simulink model "SecRwLtStHdrstFwdBkwdTrgtPosSelc"  (R2018b)
settings: Solver=FixedStepDiscrete  StartTime=0.0  StopTime=10.0  FixedStep=0.01  RelTol=1e-3
undefined symbols (not defined in the file or in its folder): KeSMSw4SAcsMd21SecRwLtStHdrstFrwdBkwdPos_Val, KeSMSw4SAcsMd21SecRwLtStHdrstFrwdBkwdPosMax_Val, KeSMSw4SAcsMd21SecRwLtStHdrstFrwdBkwdPosMin_Val, KeSMSw4SAcsMd22SecRwLtStHdrstFrwdBkwdPos_Val, KeSMSw4SAcsMd22SecRwLtStHdrstFrwdBkwdPosMax_Val, KeSMSw4SAcsMd22SecRwLtStHdrstFrwdBkwdPosMin_Val, KeSMSw4SAcsMd25SecRwLtStHdrstFrwdBkwdPos_Val, KeSMSw4SAcsMd25SecRwLtStHdrstFrwdBkwdPosMax_Val, KeSMSw4SAcsMd25SecRwLtStHdrstFrwdBkwdPosMin_Val, KeSMSw4SAcsMd26SecRwLtStHdrstFrwdBkwdPos_Val, KeSMSw4SAcsMd26SecRwLtStHdrstFrwdBkwdPosMax_Val, KeSMSw4SAcsMd26SecRwLtStHdrstFrwdBkwdPosMin_Val, KeSMSw4sLyingMDSecRwLtStHdrstFrwdBkwdnwdPos_160_Val, KeSMSw4sLyingMDSecRwLtStHdrstFrwdBkwdnwdPos_165_Val, KeSMSw4sLyingMDSecRwLtStHdrstFrwdBkwdnwdPos_170_Val, KeSMSw4sLyingMDSecRwLtStHdrstFrwdBkwdnwdPos_175_Val, KeSMSw4sLyingMDSecRwLtStHdrstFrwdBkwdnwdPos_180_Val, KeSMSw4sLyingMDSecRwLtStHdrstFrwdBkwdnwdPos_Below160_Val, KeSMSw4sLyingMDSecRwLtStHdrstFrwdBkwdnwdPos_Over180_Val, KeSMSw4sLyingMDSecRwLtStHdrstFrwdBkwdnwdPosMax_160_Val, KeSMSw4sLyingMDSecRwLtStHdrstFrwdBkwdnwdPosMax_165_Val, KeSMSw4sLyingMDSecRwLtStHdrstFrwdBkwdnwdPosMax_170_Val, KeSMSw4sLyingMDSecRwLtStHdrstFrwdBkwdnwdPosMax_175_Val, KeSMSw4sLyingMDSecRwLtStHdrstFrwdBkwdnwdPosMax_180_Val, KeSMSw4sLyingMDSecRwLtStHdrstFrwdBkwdnwdPosMax_Below160_Val, KeSMSw4sLyingMDSecRwLtStHdrstFrwdBkwdnwdPosMax_Over180_Val, KeSMSw4sLyingMDSecRwLtStHdrstFrwdBkwdnwdPosMin_160_Val, KeSMSw4sLyingMDSecRwLtStHdrstFrwdBkwdnwdPosMin_165_Val, KeSMSw4sLyingMDSecRwLtStHdrstFrwdBkwdnwdPosMin_170_Val, KeSMSw4sLyingMDSecRwLtStHdrstFrwdBkwdnwdPosMin_175_Val, KeSMSw4sLyingMDSecRwLtStHdrstFrwdBkwdnwdPosMin_180_Val, KeSMSw4sLyingMDSecRwLtStHdrstFrwdBkwdnwdPosMin_Below160_Val, KeSMSw4sLyingMDSecRwLtStHdrstFrwdBkwdnwdPosMin_Over180_Val, KeSMSw4sRecoveryMDSecRwLtStHdrstFrwdBkwdPos_160_Val, KeSMSw4sRecoveryMDSecRwLtStHdrstFrwdBkwdPos_165_Val, KeSMSw4sRecoveryMDSecRwLtStHdrstFrwdBkwdPos_170_Val, KeSMSw4sRecoveryMDSecRwLtStHdrstFrwdBkwdPos_175_Val, KeSMSw4sRecoveryMDSecRwLtStHdrstFrwdBkwdPos_180_Val, KeSMSw4sRecoveryMDSecRwLtStHdrstFrwdBkwdPos_Below160_Val, KeSMSw4sRecoveryMDSecRwLtStHdrstFrwdBkwdPos_Over180_Val, KeSMSw4sRecoveryMDSecRwLtStHdrstFrwdBkwdPosMax_160_Val, KeSMSw4sRecoveryMDSecRwLtStHdrstFrwdBkwdPosMax_165_Val, KeSMSw4sRecoveryMDSecRwLtStHdrstFrwdBkwdPosMax_170_Val, KeSMSw4sRecoveryMDSecRwLtStHdrstFrwdBkwdPosMax_175_Val, KeSMSw4sRecoveryMDSecRwLtStHdrstFrwdBkwdPosMax_180_Val, KeSMSw4sRecoveryMDSecRwLtStHdrstFrwdBkwdPosMax_Below160_Val, KeSMSw4sRecoveryMDSecRwLtStHdrstFrwdBkwdPosMax_Over180_Val, KeSMSw4sRecoveryMDSecRwLtStHdrstFrwdBkwdPosMin_160_Val, KeSMSw4sRecoveryMDSecRwLtStHdrstFrwdBkwdPosMin_165_Val, KeSMSw4sRecoveryMDSecRwLtStHdrstFrwdBkwdPosMin_170_Val, KeSMSw4sRecoveryMDSecRwLtStHdrstFrwdBkwdPosMin_175_Val, KeSMSw4sRecoveryMDSecRwLtStHdrstFrwdBkwdPosMin_180_Val, KeSMSw4sRecoveryMDSecRwLtStHdrstFrwdBkwdPosMin_Below160_Val, KeSMSw4sRecoveryMDSecRwLtStHdrstFrwdBkwdPosMin_Over180_Val, KeSMSw4sVIPMDSecRwLtStHdrstFrwdBkwdPos_160_Val, KeSMSw4sVIPMDSecRwLtStHdrstFrwdBkwdPos_165_Val, KeSMSw4sVIPMDSecRwLtStHdrstFrwdBkwdPos_170_Val, KeSMSw4sVIPMDSecRwLtStHdrstFrwdBkwdPos_175_Val, KeSMSw4sVIPMDSecRwLtStHdrstFrwdBkwdPos_180_Val, KeSMSw4sVIPMDSecRwLtStHdrstFrwdBkwdPos_Below160_Val ... (+15)
libraries: TrgtPosSelcLib x7
settings Model: ModifiedHistory=2023.8.1 V2.0.0 CR401790 增加模式21-26  Creator=sn2xws  LastModifiedBy=sn2xws
settings DataIOCC: SaveFormat=StructureWithTime
settings OptimizationCC: DefaultParameterBehavior=Inlined  EnhancedBackFolding=on  PassReuseOutputArgsAs=Individual arguments  ZeroExternalMemoryAtStartup=off  ZeroInternalMemoryAtStartup=off  OptimizeBlockOrder=speed  DifferentSizesBufferReuse=on  OptimizationCustomize=off
settings DebuggingCC: ParameterTunabilityLossMsg=error
settings ModelReferenceCC: ModelReferenceNumInstancesAllowed=Single
settings SFSimCC: MATLABDynamicMemAlloc=off
settings RTWCC: SystemTargetFile=autosar.tlc  GenCodeOnly=on  TemplateMakefile=ert_default_tmf  Description=AUTOSAR  GenerateReport=on  IncludeHyperlinkInReport=on  LaunchReport=on  GenerateTraceInfo=on  GenerateTraceReport=on  GenerateTraceReportSl=on  GenerateTraceReportSf=on  GenerateTraceReportEml=on  GenerateCodeMetricsReport=on
settings CodeAppCC: ForceParamTrailComments=on  IgnoreCustomStorageClasses=off  OperatorAnnotations=on  SimulinkDataObjDesc=on  SFDataObjDesc=on  InsertBlockDesc=on
settings STFCustomTargetCC: TargetLangStandard=C99 (ISO)  MultiwordLength=256  ParMdlRefBuildCompliant=on  CompOptLevelCompliant=on  IncludeMdlTerminateFcn=off  CombineOutputUpdateFcns=on  SuppressErrorStatus=on  ERTCustomFileBanners=on  SupportNonFinite=off  SupportComplex=off  SupportContinuousTime=off  SupportNonInlinedSFcns=off  RemoveResetFunc=on  MATLABClassNameForMDSCustomization=Simulink.SoftwareTarget.ERTCustomization  AutosarCompliant=on  UseToolchainInfoCompliant=on  LookupTableObjectStructAxisOrder=2,1,3,4,...  LUTObjectStructOrderEvenSpacing=Size,Table,Breakpoints  SystemTargetFile=autosar.tlc
settings ERTTargetCC: TargetLangStandard=C99 (ISO)  ConcurrentExecutionCompliant=off  IncludeMdlTerminateFcn=off  SuppressErrorStatus=on  SupportNonFinite=off  SupportComplex=off  ModelStepFunctionPrototypeControlCompliant=off  CPPClassGenCompliant=off  AutosarCompliant=on  LookupTableObjectStructAxisOrder=2,1,3,4,...  LUTObjectStructOrderEvenSpacing=Size,Table,Breakpoints  InlinedParameterPlacement=NonHierarchical  ERTCustomFileTemplate=example_file_process.tlc  ERTFilePackagingFormat=Compact

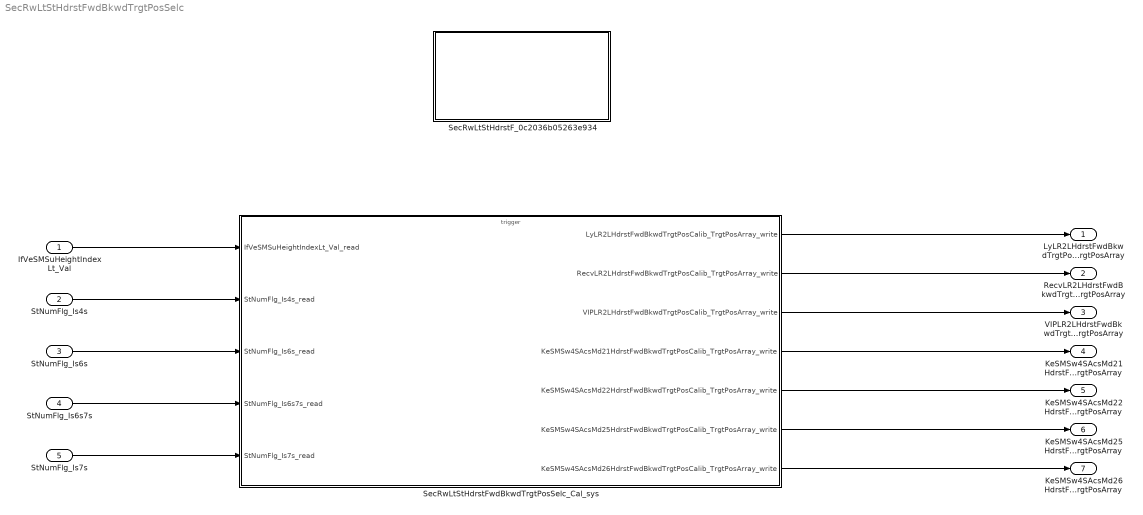
== system SecRwLtStHdrstFwdBkwdTrgtPosSelc ==
  IfVeSMSuHeightIndexLt_Val : Inport  Description=|  OutDataTypeStr=uint8  PortDimensions=1
      | 0：under 160
      | 1：160
      | 2：165
      | 3：170
      | 4：175
      | 5：180
      | 6：over 180
  StNumFlg_Is4s : Inport  Port=2  OutDataTypeStr=boolean  PortDimensions=1
  StNumFlg_Is6s : Inport  Port=3  OutDataTypeStr=boolean  PortDimensions=1
  StNumFlg_Is6s7s : Inport  Port=4  OutDataTypeStr=boolean  PortDimensions=1
  StNumFlg_Is7s : Inport  Port=5  OutDataTypeStr=boolean  PortDimensions=1
  SecRwLtStHdrstF_0c2036b05263e934 : Subsystem
  SecRwLtStHdrstFwdBkwdTrgtPosSelc_Cal_sys : Subsystem
  LyLR2LHdrstFwdBkwdTrgtPosCalib_TrgtPosArray : Outport  Description=|  OutDataTypeStr=uint16  PortDimensions=3
      | 0:Pos
      | 1:Max
      | 2:Min
  RecvLR2LHdrstFwdBkwdTrgtPosCalib_TrgtPosArray : Outport  Description=|  Port=2  OutDataTypeStr=uint16  PortDimensions=3
      | 0:Pos
      | 1:Max
      | 2:Min
  VIPLR2LHdrstFwdBkwdTrgtPosCalib_TrgtPosArray : Outport  Description=|  Port=3  OutDataTypeStr=uint16  PortDimensions=3
      | 0:Pos
      | 1:Max
      | 2:Min
  KeSMSw4SAcsMd21HdrstFwdBkwdTrgtPosCalib_TrgtPosArray : Outport  Description=|  Port=4  OutDataTypeStr=uint16  PortDimensions=3
      | 0:Pos
      | 1:Max
      | 2:Min
  KeSMSw4SAcsMd22HdrstFwdBkwdTrgtPosCalib_TrgtPosArray : Outport  Description=|  Port=5  OutDataTypeStr=uint16  PortDimensions=3
      | 0:Pos
      | 1:Max
      | 2:Min
  KeSMSw4SAcsMd25HdrstFwdBkwdTrgtPosCalib_TrgtPosArray : Outport  Description=|  Port=6  OutDataTypeStr=uint16  PortDimensions=3
      | 0:Pos
      | 1:Max
      | 2:Min
  KeSMSw4SAcsMd26HdrstFwdBkwdTrgtPosCalib_TrgtPosArray : Outport  Description=|  Port=7  OutDataTypeStr=uint16  PortDimensions=3
      | 0:Pos
      | 1:Max
      | 2:Min
  wires:
  IfVeSMSuHeightIndexLt_Val/1 -> SecRwLtStHdrstFwdBkwdTrgtPosSelc_Cal_sys/1(IfVeSMSuHeightIndexLt_Val_read)
  StNumFlg_Is4s/1 -> SecRwLtStHdrstFwdBkwdTrgtPosSelc_Cal_sys/2(StNumFlg_Is4s_read)
  StNumFlg_Is6s/1 -> SecRwLtStHdrstFwdBkwdTrgtPosSelc_Cal_sys/3(StNumFlg_Is6s_read)
  StNumFlg_Is6s7s/1 -> SecRwLtStHdrstFwdBkwdTrgtPosSelc_Cal_sys/4(StNumFlg_Is6s7s_read)
  StNumFlg_Is7s/1 -> SecRwLtStHdrstFwdBkwdTrgtPosSelc_Cal_sys/5(StNumFlg_Is7s_read)
  SecRwLtStHdrstFwdBkwdTrgtPosSelc_Cal_sys/1(LyLR2LHdrstFwdBkwdTrgtPosCalib_TrgtPosArray_write) -> LyLR2LHdrstFwdBkwdTrgtPosCalib_TrgtPosArray/1
  SecRwLtStHdrstFwdBkwdTrgtPosSelc_Cal_sys/2(RecvLR2LHdrstFwdBkwdTrgtPosCalib_TrgtPosArray_write) -> RecvLR2LHdrstFwdBkwdTrgtPosCalib_TrgtPosArray/1
  SecRwLtStHdrstFwdBkwdTrgtPosSelc_Cal_sys/3(VIPLR2LHdrstFwdBkwdTrgtPosCalib_TrgtPosArray_write) -> VIPLR2LHdrstFwdBkwdTrgtPosCalib_TrgtPosArray/1
  SecRwLtStHdrstFwdBkwdTrgtPosSelc_Cal_sys/4(KeSMSw4SAcsMd21HdrstFwdBkwdTrgtPosCalib_TrgtPosArray_write) -> KeSMSw4SAcsMd21HdrstFwdBkwdTrgtPosCalib_TrgtPosArray/1
  SecRwLtStHdrstFwdBkwdTrgtPosSelc_Cal_sys/5(KeSMSw4SAcsMd22HdrstFwdBkwdTrgtPosCalib_TrgtPosArray_write) -> KeSMSw4SAcsMd22HdrstFwdBkwdTrgtPosCalib_TrgtPosArray/1
  SecRwLtStHdrstFwdBkwdTrgtPosSelc_Cal_sys/6(KeSMSw4SAcsMd25HdrstFwdBkwdTrgtPosCalib_TrgtPosArray_write) -> KeSMSw4SAcsMd25HdrstFwdBkwdTrgtPosCalib_TrgtPosArray/1
  SecRwLtStHdrstFwdBkwdTrgtPosSelc_Cal_sys/7(KeSMSw4SAcsMd26HdrstFwdBkwdTrgtPosCalib_TrgtPosArray_write) -> KeSMSw4SAcsMd26HdrstFwdBkwdTrgtPosCalib_TrgtPosArray/1

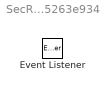
== system SecRwLtStHdrstFwdBkwdTrgtPosSelc/SecRwLtStHdrstF_0c2036b05263e934 ==
  Event Listener : EventListener  EventName=reset

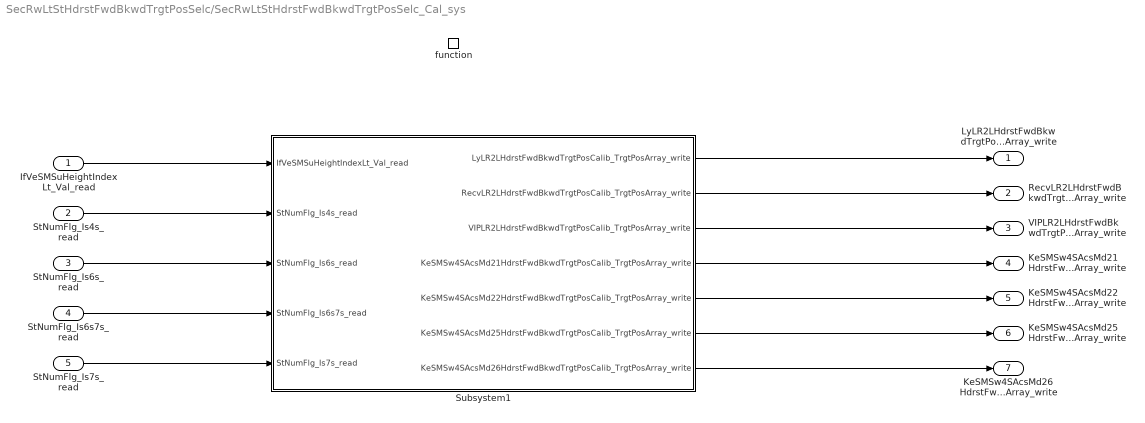
== system SecRwLtStHdrstFwdBkwdTrgtPosSelc/SecRwLtStHdrstFwdBkwdTrgtPosSelc_Cal_sys ==
  IfVeSMSuHeightIndexLt_Val_read : Inport
  StNumFlg_Is4s_read : Inport  Port=2
  StNumFlg_Is6s_read : Inport  Port=3
  StNumFlg_Is6s7s_read : Inport  Port=4
  StNumFlg_Is7s_read : Inport  Port=5
  function : TriggerPort  TriggerType=function-call  IsSimulinkFunction=on  FunctionName=SecRwLtStHdrstFwdBkwdTrgtPosSelc_Cal  VariantControl=(inherit)
  Subsystem1 : Subsystem
  LyLR2LHdrstFwdBkwdTrgtPosCalib_TrgtPosArray_write : Outport
      settings: EnsureOutportIsVirtual=on
  RecvLR2LHdrstFwdBkwdTrgtPosCalib_TrgtPosArray_write : Outport  Port=2
      settings: EnsureOutportIsVirtual=on
  VIPLR2LHdrstFwdBkwdTrgtPosCalib_TrgtPosArray_write : Outport  Port=3
      settings: EnsureOutportIsVirtual=on
  KeSMSw4SAcsMd21HdrstFwdBkwdTrgtPosCalib_TrgtPosArray_write : Outport  Port=4
      settings: EnsureOutportIsVirtual=on
  KeSMSw4SAcsMd22HdrstFwdBkwdTrgtPosCalib_TrgtPosArray_write : Outport  Port=5
      settings: EnsureOutportIsVirtual=on
  KeSMSw4SAcsMd25HdrstFwdBkwdTrgtPosCalib_TrgtPosArray_write : Outport  Port=6
      settings: EnsureOutportIsVirtual=on
  KeSMSw4SAcsMd26HdrstFwdBkwdTrgtPosCalib_TrgtPosArray_write : Outport  Port=7
      settings: EnsureOutportIsVirtual=on
  wires:
  Subsystem1/1(LyLR2LHdrstFwdBkwdTrgtPosCalib_TrgtPosArray_write) -> LyLR2LHdrstFwdBkwdTrgtPosCalib_TrgtPosArray_write/1
  Subsystem1/2(RecvLR2LHdrstFwdBkwdTrgtPosCalib_TrgtPosArray_write) -> RecvLR2LHdrstFwdBkwdTrgtPosCalib_TrgtPosArray_write/1
  Subsystem1/3(VIPLR2LHdrstFwdBkwdTrgtPosCalib_TrgtPosArray_write) -> VIPLR2LHdrstFwdBkwdTrgtPosCalib_TrgtPosArray_write/1
  Subsystem1/4(KeSMSw4SAcsMd21HdrstFwdBkwdTrgtPosCalib_TrgtPosArray_write) -> KeSMSw4SAcsMd21HdrstFwdBkwdTrgtPosCalib_TrgtPosArray_write/1
  Subsystem1/5(KeSMSw4SAcsMd22HdrstFwdBkwdTrgtPosCalib_TrgtPosArray_write) -> KeSMSw4SAcsMd22HdrstFwdBkwdTrgtPosCalib_TrgtPosArray_write/1
  Subsystem1/6(KeSMSw4SAcsMd25HdrstFwdBkwdTrgtPosCalib_TrgtPosArray_write) -> KeSMSw4SAcsMd25HdrstFwdBkwdTrgtPosCalib_TrgtPosArray_write/1
  Subsystem1/7(KeSMSw4SAcsMd26HdrstFwdBkwdTrgtPosCalib_TrgtPosArray_write) -> KeSMSw4SAcsMd26HdrstFwdBkwdTrgtPosCalib_TrgtPosArray_write/1
  StNumFlg_Is4s_read/1 -> Subsystem1/2(StNumFlg_Is4s_read)
  StNumFlg_Is6s_read/1 -> Subsystem1/3(StNumFlg_Is6s_read)
  IfVeSMSuHeightIndexLt_Val_read/1 -> Subsystem1/1(IfVeSMSuHeightIndexLt_Val_read)
  StNumFlg_Is6s7s_read/1 -> Subsystem1/4(StNumFlg_Is6s7s_read)
  StNumFlg_Is7s_read/1 -> Subsystem1/5(StNumFlg_Is7s_read)

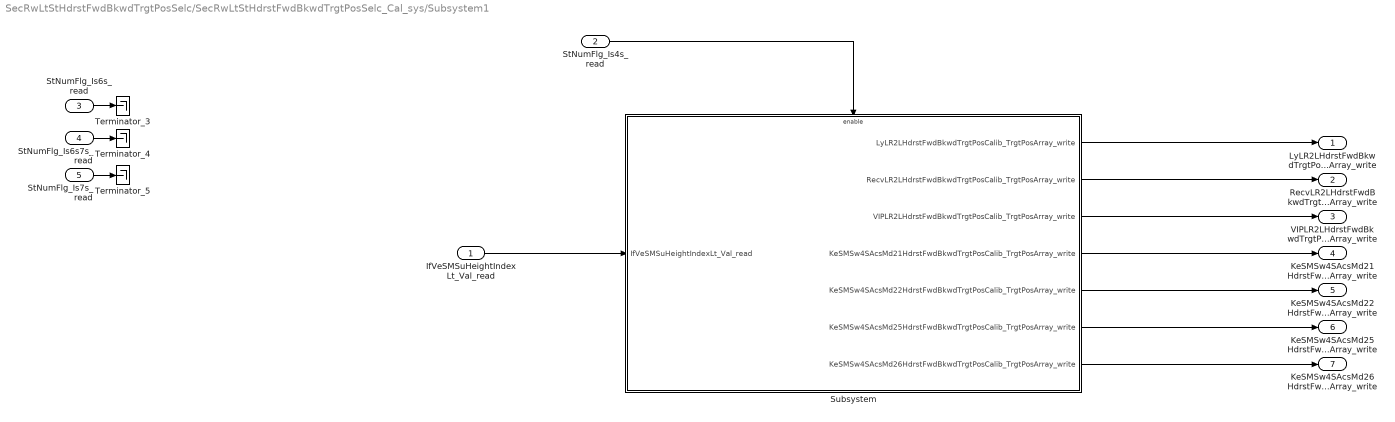
== system SecRwLtStHdrstFwdBkwdTrgtPosSelc/SecRwLtStHdrstFwdBkwdTrgtPosSelc_Cal_sys/Subsystem1 ==
  IfVeSMSuHeightIndexLt_Val_read : Inport
  StNumFlg_Is4s_read : Inport  Port=2
  StNumFlg_Is6s_read : Inport  Port=3
  StNumFlg_Is6s7s_read : Inport  Port=4
  StNumFlg_Is7s_read : Inport  Port=5
  Subsystem : Subsystem
  Terminator_3 : Terminator
  Terminator_4 : Terminator
  Terminator_5 : Terminator
  LyLR2LHdrstFwdBkwdTrgtPosCalib_TrgtPosArray_write : Outport
      settings: EnsureOutportIsVirtual=on
  RecvLR2LHdrstFwdBkwdTrgtPosCalib_TrgtPosArray_write : Outport  Port=2
      settings: EnsureOutportIsVirtual=on
  VIPLR2LHdrstFwdBkwdTrgtPosCalib_TrgtPosArray_write : Outport  Port=3
      settings: EnsureOutportIsVirtual=on
  KeSMSw4SAcsMd21HdrstFwdBkwdTrgtPosCalib_TrgtPosArray_write : Outport  Port=4
      settings: EnsureOutportIsVirtual=on
  KeSMSw4SAcsMd22HdrstFwdBkwdTrgtPosCalib_TrgtPosArray_write : Outport  Port=5
      settings: EnsureOutportIsVirtual=on
  KeSMSw4SAcsMd25HdrstFwdBkwdTrgtPosCalib_TrgtPosArray_write : Outport  Port=6
      settings: EnsureOutportIsVirtual=on
  KeSMSw4SAcsMd26HdrstFwdBkwdTrgtPosCalib_TrgtPosArray_write : Outport  Port=7
      settings: EnsureOutportIsVirtual=on
  wires:
  Subsystem/2(RecvLR2LHdrstFwdBkwdTrgtPosCalib_TrgtPosArray_write) -> RecvLR2LHdrstFwdBkwdTrgtPosCalib_TrgtPosArray_write/1
  Subsystem/1(LyLR2LHdrstFwdBkwdTrgtPosCalib_TrgtPosArray_write) -> LyLR2LHdrstFwdBkwdTrgtPosCalib_TrgtPosArray_write/1
  StNumFlg_Is4s_read/1 -> Subsystem/Enable
  IfVeSMSuHeightIndexLt_Val_read/1 -> Subsystem/1(IfVeSMSuHeightIndexLt_Val_read)
  Subsystem/3(VIPLR2LHdrstFwdBkwdTrgtPosCalib_TrgtPosArray_write) -> VIPLR2LHdrstFwdBkwdTrgtPosCalib_TrgtPosArray_write/1
  StNumFlg_Is7s_read/1 -> Terminator_5/1
  StNumFlg_Is6s7s_read/1 -> Terminator_4/1
  StNumFlg_Is6s_read/1 -> Terminator_3/1
  Subsystem/7(KeSMSw4SAcsMd26HdrstFwdBkwdTrgtPosCalib_TrgtPosArray_write) -> KeSMSw4SAcsMd26HdrstFwdBkwdTrgtPosCalib_TrgtPosArray_write/1
  Subsystem/6(KeSMSw4SAcsMd25HdrstFwdBkwdTrgtPosCalib_TrgtPosArray_write) -> KeSMSw4SAcsMd25HdrstFwdBkwdTrgtPosCalib_TrgtPosArray_write/1
  Subsystem/5(KeSMSw4SAcsMd22HdrstFwdBkwdTrgtPosCalib_TrgtPosArray_write) -> KeSMSw4SAcsMd22HdrstFwdBkwdTrgtPosCalib_TrgtPosArray_write/1
  Subsystem/4(KeSMSw4SAcsMd21HdrstFwdBkwdTrgtPosCalib_TrgtPosArray_write) -> KeSMSw4SAcsMd21HdrstFwdBkwdTrgtPosCalib_TrgtPosArray_write/1

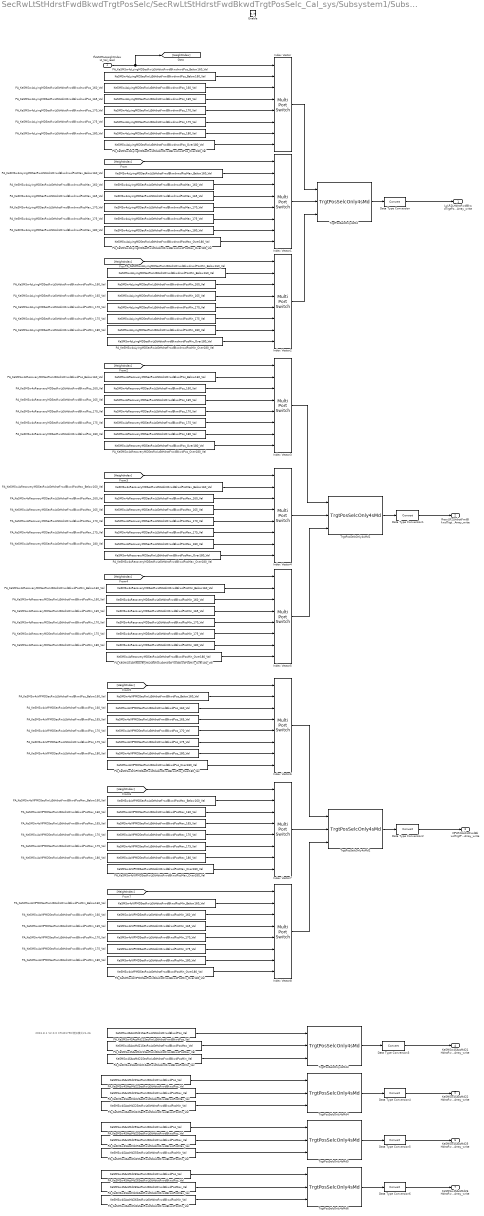
== system SecRwLtStHdrstFwdBkwdTrgtPosSelc/SecRwLtStHdrstFwdBkwdTrgtPosSelc_Cal_sys/Subsystem1/Subsystem ==
  note: 2023.8.1 V2.0.0 CR401790 增加模式21-26
  IfVeSMSuHeightIndexLt_Val_read : Inport
  Enable : EnablePort
  Data Type Conversion{,1..6} (7 alike) : DataTypeConversion
  Index Vector{,1..8} (9 alike) : MultiPortSwitch  DataPortOrder=Zero-based contiguous  Inputs=7  zeroidx=on
  PA_KeSMSw4SAcsMd21SecRwLtStHdrstFrwdBkwdPosMax_Val : Constant  Value=KeSMSw4SAcsMd21SecRwLtStHdrstFrwdBkwdPosMax_Val
  PA_KeSMSw4SAcsMd21SecRwLtStHdrstFrwdBkwdPosMin_Val : Constant  Value=KeSMSw4SAcsMd21SecRwLtStHdrstFrwdBkwdPosMin_Val
  PA_KeSMSw4SAcsMd21SecRwLtStHdrstFrwdBkwdPos_Val : Constant  Value=KeSMSw4SAcsMd21SecRwLtStHdrstFrwdBkwdPos_Val
  PA_KeSMSw4SAcsMd22SecRwLtStHdrstFrwdBkwdPosMax_Val : Constant  Value=KeSMSw4SAcsMd22SecRwLtStHdrstFrwdBkwdPosMax_Val
  PA_KeSMSw4SAcsMd22SecRwLtStHdrstFrwdBkwdPosMin_Val : Constant  Value=KeSMSw4SAcsMd22SecRwLtStHdrstFrwdBkwdPosMin_Val
  PA_KeSMSw4SAcsMd22SecRwLtStHdrstFrwdBkwdPos_Val : Constant  Value=KeSMSw4SAcsMd22SecRwLtStHdrstFrwdBkwdPos_Val
  PA_KeSMSw4SAcsMd25SecRwLtStHdrstFrwdBkwdPosMax_Val : Constant  Value=KeSMSw4SAcsMd25SecRwLtStHdrstFrwdBkwdPosMax_Val
  PA_KeSMSw4SAcsMd25SecRwLtStHdrstFrwdBkwdPosMin_Val : Constant  Value=KeSMSw4SAcsMd25SecRwLtStHdrstFrwdBkwdPosMin_Val
  PA_KeSMSw4SAcsMd25SecRwLtStHdrstFrwdBkwdPos_Val : Constant  Value=KeSMSw4SAcsMd25SecRwLtStHdrstFrwdBkwdPos_Val
  PA_KeSMSw4SAcsMd26SecRwLtStHdrstFrwdBkwdPosMax_Val : Constant  Value=KeSMSw4SAcsMd26SecRwLtStHdrstFrwdBkwdPosMax_Val
  PA_KeSMSw4SAcsMd26SecRwLtStHdrstFrwdBkwdPosMin_Val : Constant  Value=KeSMSw4SAcsMd26SecRwLtStHdrstFrwdBkwdPosMin_Val
  PA_KeSMSw4SAcsMd26SecRwLtStHdrstFrwdBkwdPos_Val : Constant  Value=KeSMSw4SAcsMd26SecRwLtStHdrstFrwdBkwdPos_Val
  PA_KeSMSw4sLyingMDSecRwLtStHdrstFrwdBkwdnwdPosMax_160_Val : Constant  Value=KeSMSw4sLyingMDSecRwLtStHdrstFrwdBkwdnwdPosMax_160_Val
  PA_KeSMSw4sLyingMDSecRwLtStHdrstFrwdBkwdnwdPosMax_165_Val : Constant  Value=KeSMSw4sLyingMDSecRwLtStHdrstFrwdBkwdnwdPosMax_165_Val
  PA_KeSMSw4sLyingMDSecRwLtStHdrstFrwdBkwdnwdPosMax_170_Val : Constant  Value=KeSMSw4sLyingMDSecRwLtStHdrstFrwdBkwdnwdPosMax_170_Val
  PA_KeSMSw4sLyingMDSecRwLtStHdrstFrwdBkwdnwdPosMax_175_Val : Constant  Value=KeSMSw4sLyingMDSecRwLtStHdrstFrwdBkwdnwdPosMax_175_Val
  PA_KeSMSw4sLyingMDSecRwLtStHdrstFrwdBkwdnwdPosMax_180_Val : Constant  Value=KeSMSw4sLyingMDSecRwLtStHdrstFrwdBkwdnwdPosMax_180_Val
  PA_KeSMSw4sLyingMDSecRwLtStHdrstFrwdBkwdnwdPosMax_Below160_Val : Constant  Value=KeSMSw4sLyingMDSecRwLtStHdrstFrwdBkwdnwdPosMax_Below160_Val
  PA_KeSMSw4sLyingMDSecRwLtStHdrstFrwdBkwdnwdPosMax_Over180_Val : Constant  Value=KeSMSw4sLyingMDSecRwLtStHdrstFrwdBkwdnwdPosMax_Over180_Val
  PA_KeSMSw4sLyingMDSecRwLtStHdrstFrwdBkwdnwdPosMin_160_Val : Constant  Value=KeSMSw4sLyingMDSecRwLtStHdrstFrwdBkwdnwdPosMin_160_Val
  PA_KeSMSw4sLyingMDSecRwLtStHdrstFrwdBkwdnwdPosMin_165_Val : Constant  Value=KeSMSw4sLyingMDSecRwLtStHdrstFrwdBkwdnwdPosMin_165_Val
  PA_KeSMSw4sLyingMDSecRwLtStHdrstFrwdBkwdnwdPosMin_170_Val : Constant  Value=KeSMSw4sLyingMDSecRwLtStHdrstFrwdBkwdnwdPosMin_170_Val
  PA_KeSMSw4sLyingMDSecRwLtStHdrstFrwdBkwdnwdPosMin_175_Val : Constant  Value=KeSMSw4sLyingMDSecRwLtStHdrstFrwdBkwdnwdPosMin_175_Val
  PA_KeSMSw4sLyingMDSecRwLtStHdrstFrwdBkwdnwdPosMin_180_Val : Constant  Value=KeSMSw4sLyingMDSecRwLtStHdrstFrwdBkwdnwdPosMin_180_Val
  PA_KeSMSw4sLyingMDSecRwLtStHdrstFrwdBkwdnwdPosMin_Below160_Val : Constant  Value=KeSMSw4sLyingMDSecRwLtStHdrstFrwdBkwdnwdPosMin_Below160_Val
  PA_KeSMSw4sLyingMDSecRwLtStHdrstFrwdBkwdnwdPosMin_Over180_Val : Constant  Value=KeSMSw4sLyingMDSecRwLtStHdrstFrwdBkwdnwdPosMin_Over180_Val
  PA_KeSMSw4sLyingMDSecRwLtStHdrstFrwdBkwdnwdPos_160_Val : Constant  Value=KeSMSw4sLyingMDSecRwLtStHdrstFrwdBkwdnwdPos_160_Val
  PA_KeSMSw4sLyingMDSecRwLtStHdrstFrwdBkwdnwdPos_165_Val : Constant  Value=KeSMSw4sLyingMDSecRwLtStHdrstFrwdBkwdnwdPos_165_Val
  PA_KeSMSw4sLyingMDSecRwLtStHdrstFrwdBkwdnwdPos_170_Val : Constant  Value=KeSMSw4sLyingMDSecRwLtStHdrstFrwdBkwdnwdPos_170_Val
  PA_KeSMSw4sLyingMDSecRwLtStHdrstFrwdBkwdnwdPos_175_Val : Constant  Value=KeSMSw4sLyingMDSecRwLtStHdrstFrwdBkwdnwdPos_175_Val
  PA_KeSMSw4sLyingMDSecRwLtStHdrstFrwdBkwdnwdPos_180_Val : Constant  Value=KeSMSw4sLyingMDSecRwLtStHdrstFrwdBkwdnwdPos_180_Val
  PA_KeSMSw4sLyingMDSecRwLtStHdrstFrwdBkwdnwdPos_Below160_Val : Constant  Value=KeSMSw4sLyingMDSecRwLtStHdrstFrwdBkwdnwdPos_Below160_Val
  PA_KeSMSw4sLyingMDSecRwLtStHdrstFrwdBkwdnwdPos_Over180_Val : Constant  Value=KeSMSw4sLyingMDSecRwLtStHdrstFrwdBkwdnwdPos_Over180_Val
  PA_KeSMSw4sRecoveryMDSecRwLtStHdrstFrwdBkwdPosMax_160_Val : Constant  Value=KeSMSw4sRecoveryMDSecRwLtStHdrstFrwdBkwdPosMax_160_Val
  PA_KeSMSw4sRecoveryMDSecRwLtStHdrstFrwdBkwdPosMax_165_Val : Constant  Value=KeSMSw4sRecoveryMDSecRwLtStHdrstFrwdBkwdPosMax_165_Val
  PA_KeSMSw4sRecoveryMDSecRwLtStHdrstFrwdBkwdPosMax_170_Val : Constant  Value=KeSMSw4sRecoveryMDSecRwLtStHdrstFrwdBkwdPosMax_170_Val
  PA_KeSMSw4sRecoveryMDSecRwLtStHdrstFrwdBkwdPosMax_175_Val : Constant  Value=KeSMSw4sRecoveryMDSecRwLtStHdrstFrwdBkwdPosMax_175_Val
  PA_KeSMSw4sRecoveryMDSecRwLtStHdrstFrwdBkwdPosMax_180_Val : Constant  Value=KeSMSw4sRecoveryMDSecRwLtStHdrstFrwdBkwdPosMax_180_Val
  PA_KeSMSw4sRecoveryMDSecRwLtStHdrstFrwdBkwdPosMax_Below160_Val : Constant  Value=KeSMSw4sRecoveryMDSecRwLtStHdrstFrwdBkwdPosMax_Below160_Val
  PA_KeSMSw4sRecoveryMDSecRwLtStHdrstFrwdBkwdPosMax_Over180_Val : Constant  Value=KeSMSw4sRecoveryMDSecRwLtStHdrstFrwdBkwdPosMax_Over180_Val
  PA_KeSMSw4sRecoveryMDSecRwLtStHdrstFrwdBkwdPosMin_160_Val : Constant  Value=KeSMSw4sRecoveryMDSecRwLtStHdrstFrwdBkwdPosMin_160_Val
  PA_KeSMSw4sRecoveryMDSecRwLtStHdrstFrwdBkwdPosMin_165_Val : Constant  Value=KeSMSw4sRecoveryMDSecRwLtStHdrstFrwdBkwdPosMin_165_Val
  PA_KeSMSw4sRecoveryMDSecRwLtStHdrstFrwdBkwdPosMin_170_Val : Constant  Value=KeSMSw4sRecoveryMDSecRwLtStHdrstFrwdBkwdPosMin_170_Val
  PA_KeSMSw4sRecoveryMDSecRwLtStHdrstFrwdBkwdPosMin_175_Val : Constant  Value=KeSMSw4sRecoveryMDSecRwLtStHdrstFrwdBkwdPosMin_175_Val
  PA_KeSMSw4sRecoveryMDSecRwLtStHdrstFrwdBkwdPosMin_180_Val : Constant  Value=KeSMSw4sRecoveryMDSecRwLtStHdrstFrwdBkwdPosMin_180_Val
  PA_KeSMSw4sRecoveryMDSecRwLtStHdrstFrwdBkwdPosMin_Below160_Val : Constant  Value=KeSMSw4sRecoveryMDSecRwLtStHdrstFrwdBkwdPosMin_Below160_Val
  PA_KeSMSw4sRecoveryMDSecRwLtStHdrstFrwdBkwdPosMin_Over180_Val : Constant  Value=KeSMSw4sRecoveryMDSecRwLtStHdrstFrwdBkwdPosMin_Over180_Val
  PA_KeSMSw4sRecoveryMDSecRwLtStHdrstFrwdBkwdPos_160_Val : Constant  Value=KeSMSw4sRecoveryMDSecRwLtStHdrstFrwdBkwdPos_160_Val
  PA_KeSMSw4sRecoveryMDSecRwLtStHdrstFrwdBkwdPos_165_Val : Constant  Value=KeSMSw4sRecoveryMDSecRwLtStHdrstFrwdBkwdPos_165_Val
  PA_KeSMSw4sRecoveryMDSecRwLtStHdrstFrwdBkwdPos_170_Val : Constant  Value=KeSMSw4sRecoveryMDSecRwLtStHdrstFrwdBkwdPos_170_Val
  PA_KeSMSw4sRecoveryMDSecRwLtStHdrstFrwdBkwdPos_175_Val : Constant  Value=KeSMSw4sRecoveryMDSecRwLtStHdrstFrwdBkwdPos_175_Val
  PA_KeSMSw4sRecoveryMDSecRwLtStHdrstFrwdBkwdPos_180_Val : Constant  Value=KeSMSw4sRecoveryMDSecRwLtStHdrstFrwdBkwdPos_180_Val
  PA_KeSMSw4sRecoveryMDSecRwLtStHdrstFrwdBkwdPos_Below160_Val : Constant  Value=KeSMSw4sRecoveryMDSecRwLtStHdrstFrwdBkwdPos_Below160_Val
  PA_KeSMSw4sRecoveryMDSecRwLtStHdrstFrwdBkwdPos_Over180_Val : Constant  Value=KeSMSw4sRecoveryMDSecRwLtStHdrstFrwdBkwdPos_Over180_Val
  PA_KeSMSw4sVIPMDSecRwLtStHdrstFrwdBkwdPosMax_160_Val : Constant  Value=KeSMSw4sVIPMDSecRwLtStHdrstFrwdBkwdPosMax_160_Val
  PA_KeSMSw4sVIPMDSecRwLtStHdrstFrwdBkwdPosMax_165_Val : Constant  Value=KeSMSw4sVIPMDSecRwLtStHdrstFrwdBkwdPosMax_165_Val
  PA_KeSMSw4sVIPMDSecRwLtStHdrstFrwdBkwdPosMax_170_Val : Constant  Value=KeSMSw4sVIPMDSecRwLtStHdrstFrwdBkwdPosMax_170_Val
  PA_KeSMSw4sVIPMDSecRwLtStHdrstFrwdBkwdPosMax_175_Val : Constant  Value=KeSMSw4sVIPMDSecRwLtStHdrstFrwdBkwdPosMax_175_Val
  PA_KeSMSw4sVIPMDSecRwLtStHdrstFrwdBkwdPosMax_180_Val : Constant  Value=KeSMSw4sVIPMDSecRwLtStHdrstFrwdBkwdPosMax_180_Val
  PA_KeSMSw4sVIPMDSecRwLtStHdrstFrwdBkwdPosMax_Below160_Val : Constant  Value=KeSMSw4sVIPMDSecRwLtStHdrstFrwdBkwdPosMax_Below160_Val
  PA_KeSMSw4sVIPMDSecRwLtStHdrstFrwdBkwdPosMax_Over180_Val : Constant  Value=KeSMSw4sVIPMDSecRwLtStHdrstFrwdBkwdPosMax_Over180_Val
  PA_KeSMSw4sVIPMDSecRwLtStHdrstFrwdBkwdPosMin_160_Val : Constant  Value=KeSMSw4sVIPMDSecRwLtStHdrstFrwdBkwdPosMin_160_Val
  PA_KeSMSw4sVIPMDSecRwLtStHdrstFrwdBkwdPosMin_165_Val : Constant  Value=KeSMSw4sVIPMDSecRwLtStHdrstFrwdBkwdPosMin_165_Val
  PA_KeSMSw4sVIPMDSecRwLtStHdrstFrwdBkwdPosMin_170_Val : Constant  Value=KeSMSw4sVIPMDSecRwLtStHdrstFrwdBkwdPosMin_170_Val
  PA_KeSMSw4sVIPMDSecRwLtStHdrstFrwdBkwdPosMin_175_Val : Constant  Value=KeSMSw4sVIPMDSecRwLtStHdrstFrwdBkwdPosMin_175_Val
  PA_KeSMSw4sVIPMDSecRwLtStHdrstFrwdBkwdPosMin_180_Val : Constant  Value=KeSMSw4sVIPMDSecRwLtStHdrstFrwdBkwdPosMin_180_Val
  PA_KeSMSw4sVIPMDSecRwLtStHdrstFrwdBkwdPosMin_Below160_Val : Constant  Value=KeSMSw4sVIPMDSecRwLtStHdrstFrwdBkwdPosMin_Below160_Val
  PA_KeSMSw4sVIPMDSecRwLtStHdrstFrwdBkwdPosMin_Over180_Val : Constant  Value=KeSMSw4sVIPMDSecRwLtStHdrstFrwdBkwdPosMin_Over180_Val
  PA_KeSMSw4sVIPMDSecRwLtStHdrstFrwdBkwdPos_160_Val : Constant  Value=KeSMSw4sVIPMDSecRwLtStHdrstFrwdBkwdPos_160_Val
  PA_KeSMSw4sVIPMDSecRwLtStHdrstFrwdBkwdPos_165_Val : Constant  Value=KeSMSw4sVIPMDSecRwLtStHdrstFrwdBkwdPos_165_Val
  PA_KeSMSw4sVIPMDSecRwLtStHdrstFrwdBkwdPos_170_Val : Constant  Value=KeSMSw4sVIPMDSecRwLtStHdrstFrwdBkwdPos_170_Val
  PA_KeSMSw4sVIPMDSecRwLtStHdrstFrwdBkwdPos_175_Val : Constant  Value=KeSMSw4sVIPMDSecRwLtStHdrstFrwdBkwdPos_175_Val
  PA_KeSMSw4sVIPMDSecRwLtStHdrstFrwdBkwdPos_180_Val : Constant  Value=KeSMSw4sVIPMDSecRwLtStHdrstFrwdBkwdPos_180_Val
  PA_KeSMSw4sVIPMDSecRwLtStHdrstFrwdBkwdPos_Below160_Val : Constant  Value=KeSMSw4sVIPMDSecRwLtStHdrstFrwdBkwdPos_Below160_Val
  PA_KeSMSw4sVIPMDSecRwLtStHdrstFrwdBkwdPos_Over180_Val : Constant  Value=KeSMSw4sVIPMDSecRwLtStHdrstFrwdBkwdPos_Over180_Val
  TrgtPosSelcOnly4sMd{,1..6} (7 alike) : TrgtPosSelcLib/TrgtPosSelcOnly4sMd  SystemSampleTime=-1
  LyLR2LHdrstFwdBkwdTrgtPosCalib_TrgtPosArray_write : Outport
  RecvLR2LHdrstFwdBkwdTrgtPosCalib_TrgtPosArray_write : Outport  Port=2
  VIPLR2LHdrstFwdBkwdTrgtPosCalib_TrgtPosArray_write : Outport  Port=3
  KeSMSw4SAcsMd21HdrstFwdBkwdTrgtPosCalib_TrgtPosArray_write : Outport  Port=4  InitialOutput=0
  KeSMSw4SAcsMd22HdrstFwdBkwdTrgtPosCalib_TrgtPosArray_write : Outport  Port=5  InitialOutput=0
  KeSMSw4SAcsMd25HdrstFwdBkwdTrgtPosCalib_TrgtPosArray_write : Outport  Port=6  InitialOutput=0
  KeSMSw4SAcsMd26HdrstFwdBkwdTrgtPosCalib_TrgtPosArray_write : Outport  Port=7  InitialOutput=0
  wires:
  TrgtPosSelcOnly4sMd1/1 -> Data Type Conversion1/1
  [HeightIndex] -> Index Vector2/1
  PA_KeSMSw4sRecoveryMDSecRwLtStHdrstFrwdBkwdPosMax_Below160_Val/1 -> Index Vector4/2
  PA_KeSMSw4sLyingMDSecRwLtStHdrstFrwdBkwdnwdPos_165_Val/1 -> Index Vector/4
  PA_KeSMSw4sRecoveryMDSecRwLtStHdrstFrwdBkwdPosMin_165_Val/1 -> Index Vector5/4
  PA_KeSMSw4sLyingMDSecRwLtStHdrstFrwdBkwdnwdPosMax_Over180_Val/1 -> Index Vector1/8
  PA_KeSMSw4sRecoveryMDSecRwLtStHdrstFrwdBkwdPos_175_Val/1 -> Index Vector3/6
  PA_KeSMSw4sLyingMDSecRwLtStHdrstFrwdBkwdnwdPosMax_170_Val/1 -> Index Vector1/5
  PA_KeSMSw4sLyingMDSecRwLtStHdrstFrwdBkwdnwdPosMax_160_Val/1 -> Index Vector1/3
  PA_KeSMSw4sLyingMDSecRwLtStHdrstFrwdBkwdnwdPosMin_180_Val/1 -> Index Vector2/7
  Index Vector/1 -> TrgtPosSelcOnly4sMd/1
  PA_KeSMSw4sLyingMDSecRwLtStHdrstFrwdBkwdnwdPosMax_165_Val/1 -> Index Vector1/4
  PA_KeSMSw4sLyingMDSecRwLtStHdrstFrwdBkwdnwdPos_Over180_Val/1 -> Index Vector/8
  PA_KeSMSw4sRecoveryMDSecRwLtStHdrstFrwdBkwdPosMax_160_Val/1 -> Index Vector4/3
  Index Vector7/1 -> TrgtPosSelcOnly4sMd2/2
  PA_KeSMSw4sVIPMDSecRwLtStHdrstFrwdBkwdPos_Over180_Val/1 -> Index Vector6/8
  PA_KeSMSw4sVIPMDSecRwLtStHdrstFrwdBkwdPosMax_Over180_Val/1 -> Index Vector7/8
  [HeightIndex] -> Index Vector1/1
  PA_KeSMSw4sLyingMDSecRwLtStHdrstFrwdBkwdnwdPosMin_Over180_Val/1 -> Index Vector2/8
  PA_KeSMSw4sRecoveryMDSecRwLtStHdrstFrwdBkwdPosMin_180_Val/1 -> Index Vector5/7
  PA_KeSMSw4sRecoveryMDSecRwLtStHdrstFrwdBkwdPos_160_Val/1 -> Index Vector3/3
  PA_KeSMSw4sLyingMDSecRwLtStHdrstFrwdBkwdnwdPos_170_Val/1 -> Index Vector/5
  PA_KeSMSw4sRecoveryMDSecRwLtStHdrstFrwdBkwdPosMin_175_Val/1 -> Index Vector5/6
  PA_KeSMSw4sRecoveryMDSecRwLtStHdrstFrwdBkwdPosMin_Below160_Val/1 -> Index Vector5/2
  PA_KeSMSw4sLyingMDSecRwLtStHdrstFrwdBkwdnwdPos_160_Val/1 -> Index Vector/3
  PA_KeSMSw4sRecoveryMDSecRwLtStHdrstFrwdBkwdPosMax_175_Val/1 -> Index Vector4/6
  PA_KeSMSw4sLyingMDSecRwLtStHdrstFrwdBkwdnwdPosMin_Below160_Val/1 -> Index Vector2/2
  PA_KeSMSw4sLyingMDSecRwLtStHdrstFrwdBkwdnwdPosMin_160_Val/1 -> Index Vector2/3
  Index Vector2/1 -> TrgtPosSelcOnly4sMd/3
  PA_KeSMSw4sRecoveryMDSecRwLtStHdrstFrwdBkwdPos_165_Val/1 -> Index Vector3/4
  IfVeSMSuHeightIndexLt_Val_read/1 -> [HeightIndex], Index Vector/1
  PA_KeSMSw4sLyingMDSecRwLtStHdrstFrwdBkwdnwdPos_180_Val/1 -> Index Vector/7
  PA_KeSMSw4sLyingMDSecRwLtStHdrstFrwdBkwdnwdPosMin_175_Val/1 -> Index Vector2/6
  PA_KeSMSw4sLyingMDSecRwLtStHdrstFrwdBkwdnwdPos_175_Val/1 -> Index Vector/6
  PA_KeSMSw4sRecoveryMDSecRwLtStHdrstFrwdBkwdPos_Below160_Val/1 -> Index Vector3/2
  PA_KeSMSw4sRecoveryMDSecRwLtStHdrstFrwdBkwdPos_Over180_Val/1 -> Index Vector3/8
  Index Vector1/1 -> TrgtPosSelcOnly4sMd/2
  [HeightIndex] -> Index Vector5/1
  TrgtPosSelcOnly4sMd2/1 -> Data Type Conversion2/1
  PA_KeSMSw4sRecoveryMDSecRwLtStHdrstFrwdBkwdPosMin_Over180_Val/1 -> Index Vector5/8
  PA_KeSMSw4sRecoveryMDSecRwLtStHdrstFrwdBkwdPosMax_165_Val/1 -> Index Vector4/4
  [HeightIndex] -> Index Vector4/1
  PA_KeSMSw4sRecoveryMDSecRwLtStHdrstFrwdBkwdPosMin_170_Val/1 -> Index Vector5/5
  PA_KeSMSw4sRecoveryMDSecRwLtStHdrstFrwdBkwdPosMax_180_Val/1 -> Index Vector4/7
  PA_KeSMSw4sLyingMDSecRwLtStHdrstFrwdBkwdnwdPosMin_165_Val/1 -> Index Vector2/4
  PA_KeSMSw4sVIPMDSecRwLtStHdrstFrwdBkwdPosMin_Over180_Val/1 -> Index Vector8/8
  PA_KeSMSw4sRecoveryMDSecRwLtStHdrstFrwdBkwdPos_170_Val/1 -> Index Vector3/5
  PA_KeSMSw4sLyingMDSecRwLtStHdrstFrwdBkwdnwdPosMax_180_Val/1 -> Index Vector1/7
  PA_KeSMSw4sRecoveryMDSecRwLtStHdrstFrwdBkwdPos_180_Val/1 -> Index Vector3/7
  PA_KeSMSw4sLyingMDSecRwLtStHdrstFrwdBkwdnwdPos_Below160_Val/1 -> Index Vector/2
  Index Vector8/1 -> TrgtPosSelcOnly4sMd2/3
  PA_KeSMSw4sRecoveryMDSecRwLtStHdrstFrwdBkwdPosMin_160_Val/1 -> Index Vector5/3
  PA_KeSMSw4sRecoveryMDSecRwLtStHdrstFrwdBkwdPosMax_Over180_Val/1 -> Index Vector4/8
  [HeightIndex] -> Index Vector7/1
  PA_KeSMSw4sLyingMDSecRwLtStHdrstFrwdBkwdnwdPosMax_Below160_Val/1 -> Index Vector1/2
  PA_KeSMSw4sLyingMDSecRwLtStHdrstFrwdBkwdnwdPosMin_170_Val/1 -> Index Vector2/5
  TrgtPosSelcOnly4sMd/1 -> Data Type Conversion/1
  [HeightIndex] -> Index Vector3/1
  [HeightIndex] -> Index Vector8/1
  Index Vector5/1 -> TrgtPosSelcOnly4sMd1/3
  [HeightIndex] -> Index Vector6/1
  Index Vector4/1 -> TrgtPosSelcOnly4sMd1/2
  Index Vector3/1 -> TrgtPosSelcOnly4sMd1/1
  Index Vector6/1 -> TrgtPosSelcOnly4sMd2/1
  PA_KeSMSw4sLyingMDSecRwLtStHdrstFrwdBkwdnwdPosMax_175_Val/1 -> Index Vector1/6
  PA_KeSMSw4sRecoveryMDSecRwLtStHdrstFrwdBkwdPosMax_170_Val/1 -> Index Vector4/5
  Data Type Conversion/1 -> LyLR2LHdrstFwdBkwdTrgtPosCalib_TrgtPosArray_write/1
  Data Type Conversion1/1 -> RecvLR2LHdrstFwdBkwdTrgtPosCalib_TrgtPosArray_write/1
  Data Type Conversion2/1 -> VIPLR2LHdrstFwdBkwdTrgtPosCalib_TrgtPosArray_write/1
  TrgtPosSelcOnly4sMd3/1 -> Data Type Conversion3/1
  TrgtPosSelcOnly4sMd6/1 -> Data Type Conversion6/1
  TrgtPosSelcOnly4sMd5/1 -> Data Type Conversion5/1
  TrgtPosSelcOnly4sMd4/1 -> Data Type Conversion4/1
  PA_KeSMSw4SAcsMd21SecRwLtStHdrstFrwdBkwdPosMax_Val/1 -> TrgtPosSelcOnly4sMd3/2
  PA_KeSMSw4SAcsMd21SecRwLtStHdrstFrwdBkwdPosMin_Val/1 -> TrgtPosSelcOnly4sMd3/3
  PA_KeSMSw4SAcsMd21SecRwLtStHdrstFrwdBkwdPos_Val/1 -> TrgtPosSelcOnly4sMd3/1
  PA_KeSMSw4SAcsMd22SecRwLtStHdrstFrwdBkwdPosMax_Val/1 -> TrgtPosSelcOnly4sMd4/2
  PA_KeSMSw4SAcsMd22SecRwLtStHdrstFrwdBkwdPosMin_Val/1 -> TrgtPosSelcOnly4sMd4/3
  PA_KeSMSw4SAcsMd22SecRwLtStHdrstFrwdBkwdPos_Val/1 -> TrgtPosSelcOnly4sMd4/1
  PA_KeSMSw4SAcsMd25SecRwLtStHdrstFrwdBkwdPosMax_Val/1 -> TrgtPosSelcOnly4sMd5/2
  PA_KeSMSw4SAcsMd25SecRwLtStHdrstFrwdBkwdPosMin_Val/1 -> TrgtPosSelcOnly4sMd5/3
  PA_KeSMSw4SAcsMd25SecRwLtStHdrstFrwdBkwdPos_Val/1 -> TrgtPosSelcOnly4sMd5/1
  PA_KeSMSw4SAcsMd26SecRwLtStHdrstFrwdBkwdPosMax_Val/1 -> TrgtPosSelcOnly4sMd6/2
  PA_KeSMSw4SAcsMd26SecRwLtStHdrstFrwdBkwdPosMin_Val/1 -> TrgtPosSelcOnly4sMd6/3
  PA_KeSMSw4SAcsMd26SecRwLtStHdrstFrwdBkwdPos_Val/1 -> TrgtPosSelcOnly4sMd6/1
  Data Type Conversion3/1 -> KeSMSw4SAcsMd21HdrstFwdBkwdTrgtPosCalib_TrgtPosArray_write/1
  Data Type Conversion4/1 -> KeSMSw4SAcsMd22HdrstFwdBkwdTrgtPosCalib_TrgtPosArray_write/1
  Data Type Conversion5/1 -> KeSMSw4SAcsMd25HdrstFwdBkwdTrgtPosCalib_TrgtPosArray_write/1
  Data Type Conversion6/1 -> KeSMSw4SAcsMd26HdrstFwdBkwdTrgtPosCalib_TrgtPosArray_write/1
  PA_KeSMSw4sVIPMDSecRwLtStHdrstFrwdBkwdPos_Below160_Val/1 -> Index Vector6/2
  PA_KeSMSw4sVIPMDSecRwLtStHdrstFrwdBkwdPos_160_Val/1 -> Index Vector6/3
  PA_KeSMSw4sVIPMDSecRwLtStHdrstFrwdBkwdPos_165_Val/1 -> Index Vector6/4
  PA_KeSMSw4sVIPMDSecRwLtStHdrstFrwdBkwdPos_170_Val/1 -> Index Vector6/5
  PA_KeSMSw4sVIPMDSecRwLtStHdrstFrwdBkwdPos_175_Val/1 -> Index Vector6/6
  PA_KeSMSw4sVIPMDSecRwLtStHdrstFrwdBkwdPos_180_Val/1 -> Index Vector6/7
  PA_KeSMSw4sVIPMDSecRwLtStHdrstFrwdBkwdPosMax_Below160_Val/1 -> Index Vector7/2
  PA_KeSMSw4sVIPMDSecRwLtStHdrstFrwdBkwdPosMax_160_Val/1 -> Index Vector7/3
  PA_KeSMSw4sVIPMDSecRwLtStHdrstFrwdBkwdPosMax_165_Val/1 -> Index Vector7/4
  PA_KeSMSw4sVIPMDSecRwLtStHdrstFrwdBkwdPosMax_170_Val/1 -> Index Vector7/5
  PA_KeSMSw4sVIPMDSecRwLtStHdrstFrwdBkwdPosMax_175_Val/1 -> Index Vector7/6
  PA_KeSMSw4sVIPMDSecRwLtStHdrstFrwdBkwdPosMax_180_Val/1 -> Index Vector7/7
  PA_KeSMSw4sVIPMDSecRwLtStHdrstFrwdBkwdPosMin_Below160_Val/1 -> Index Vector8/2
  PA_KeSMSw4sVIPMDSecRwLtStHdrstFrwdBkwdPosMin_160_Val/1 -> Index Vector8/3
  PA_KeSMSw4sVIPMDSecRwLtStHdrstFrwdBkwdPosMin_165_Val/1 -> Index Vector8/4
  PA_KeSMSw4sVIPMDSecRwLtStHdrstFrwdBkwdPosMin_170_Val/1 -> Index Vector8/5
  PA_KeSMSw4sVIPMDSecRwLtStHdrstFrwdBkwdPosMin_175_Val/1 -> Index Vector8/6
  PA_KeSMSw4sVIPMDSecRwLtStHdrstFrwdBkwdPosMin_180_Val/1 -> Index Vector8/7
